simulink model "KinematicsSolverSimscape"  (R2018b)
settings: Solver=ode3  StartTime=0.0  StopTime=3  FixedStep=0.001  RelTol=1e-3
PreLoadFcn:
  | run('Arm6Assembly_DataFile.m');
model workspace: external: MAT-File E:\SixRobotArm\Simscape_Simulation\StepFile\Arm6Assembly_DataFile.mat (data not in the file)
values from neighbouring files (symbols this model uses):
  smiData =     [Arm6SimscapeData.mat]
undefined symbols (not defined in the file or in its folder): X, Y, Z
libraries: fl_lib x187, nesl_utility x55, sm_lib x36, elec_lib x12, simulink_extras x7, simulink x6
(part 1 of 4)
settings Model: Creator=Administrator  LastModifiedBy=Jeason
settings DataIOCC: ReturnWorkspaceOutputs=on
settings ExplorerConfigSet: InternalSimMechanicsExplorerSettings="<ExplorerConfiguration><canonicalview>planar_xy</canonicalview><AnimationSetting><BasePlaybackSpeed>1.0</BasePlaybackSpeed><PlaybackSpeedFactor>0.5</PlaybackSpeedFactor></AnimationSetting><TilePanel><TileInfo><Tiles Columns=\"1\" Count=\"1\" Rows=\"1\"><Column Weight=\"1\"/><Row Weight=\"1\"/><Tile Height=\"1\" Width=\"1\" X=\"0\" Y=\"0\"/></Tiles></TileInfo><SceneInfo><SceneViewer><BGColor><R>0.60000002384185791</R><G>0.60000002384185791</G><B>0.60000002384185791</B></BGColor><Camera><DoPerspective>off</DoPerspective><Position><X>-0.504262514033846698</X><Y>0.881384571408073469</Y><Z>0.0888981961479472504</Z></Position><Center><X>0.248760542540387375</X><Y>0.293287954006147933</Y><Z>-0.20622659926582132</Z></Center><Up><X>0.445605319462419325</X><Y>0.785803061090466048</Y><Z>-0.428893283285771199</Z></Up><ViewLimDist>1</ViewLimDist><YLim>0.601033807151443056</YLim><XLim>0.667231586610430694</XLim></Camera></SceneViewer></SceneInfo></TilePanel><MechEditorPanel><Cameras/><GfxPanelCameraMap/><VideoCreator><PlaybackSpeedRatio>1.0</PlaybackSpeedRatio><FrameRate>30</FrameRate><VideoFormat>MPEG-4</VideoFormat><FrameSize>[800 600]</FrameSize></VideoCreator></MechEditorPanel></ExplorerConfiguration>"

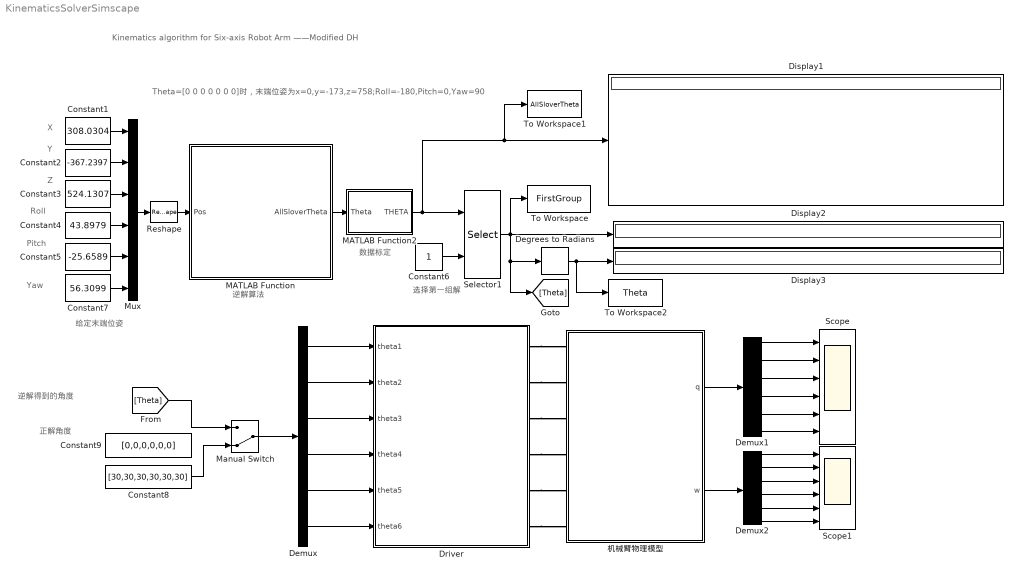
== system KinematicsSolverSimscape ==
  note: 选择第一组解
  note: 数据标定
  note: Kinematics algorithm for Six-axis Robot Arm ——Modified DH
  note: 正解角度
  note: Theta=[0 0 0 0 0 0 0]时，末端位姿为x=0,y=-173,z=758;Roll=-180,Pitch=0,Yaw=90
  note: 逆解得到的角度
  note: 逆解算法
  note: X
  note: Yaw
  note: 给定末端位姿
  note: Z
  note: Y
  note: Pitch
  note: Roll
  Constant1 : Constant  Value=308.0304
  Constant2 : Constant  Value=-367.2397
  Constant3 : Constant  Value=524.1307
  Constant4 : Constant  Value=43.8979
  Constant5 : Constant  Value=-25.6589
  Constant6 : Constant
  Constant7 : Constant  Value=56.3099
  Constant8 : Constant  Value=[30,30,30,30,30,30]
  Constant9 : Constant  Value=[0,0,0,0,0,0]
  Degrees to Radians : simulink_extras/Transformations/Degrees to Radians
  Demux : Demux  Outputs=6
  Demux1 : Demux  Outputs=6
  Demux2 : Demux  Outputs=6
  Display1 : Display
  Display2 : Display
  Display3 : Display
  Driver : Subsystem  mask{angle1=0, angle2=0, angle3=0, angle4=0, angle5=0, angle6=0}
      mask prompts: angle1 "InitTheta1(deg)"; angle2 "InitTheta2(deg)"; angle3 "InitTheta3(deg)"; angle4 "InitTheta4(deg)"; angle5 "InitTheta5(deg)"; angle6 "InitTheta6(deg)"
  MATLAB Function : MATLAB Function  TreatAsAtomicUnit=on
  MATLAB Function2 : MATLAB Function  TreatAsAtomicUnit=on
  Manual Switch : ManualSwitch  CurrentSetting=0
  Mux : Mux  Inputs=6
  Reshape : Reshape  OutputDimensionality=Customize  OutputDimensions=[1,6]
  Scope : Scope  NumInputPorts=6
  Scope1 : Scope  NumInputPorts=6
  Selector1 : Selector  NumberOfDimensions=2  InputPortWidth=10  IndexOptions=Index vector (port),Starting index (dialog)  Indices=[1 3],1  OutputSizes=1,6
  To Workspace : ToWorkspace  VariableName=FirstGroup  SampleTime=-1
      settings: MaxDataPoints=1
  To Workspace1 : ToWorkspace  VariableName=AllSloverTheta  SampleTime=-1
      settings: MaxDataPoints=1
  To Workspace2 : ToWorkspace  VariableName=Theta  SampleTime=-1
      settings: MaxDataPoints=1
  机械臂物理模型 : Subsystem
  wires:
  Constant2/1 -> Mux/2
  MATLAB Function2/1(THETA) -> To Workspace1/1, Display1/1, Selector1/1
  Constant1/1 -> Mux/1
  Demux/5 -> Driver/5(theta5)
  Constant7/1 -> Mux/6
  Manual Switch/1 -> Demux/1
  MATLAB Function/1(AllSloverTheta) -> MATLAB Function2/1(Theta)
  Demux/2 -> Driver/2(theta2)
  Mux/1 -> Reshape/1
  Constant6/1 -> Selector1/2
  Reshape/1 -> MATLAB Function/1(Pos)
  Demux/4 -> Driver/4(theta4)
  Degrees to Radians/1 -> To Workspace2/1, Display3/1
  Demux/3 -> Driver/3(theta3)
  [Theta] -> Manual Switch/1
  Selector1/1 -> To Workspace/1, [Theta], Degrees to Radians/1, Display2/1
  Constant3/1 -> Mux/3
  Demux/6 -> Driver/6(theta6)
  Constant4/1 -> Mux/4
  Constant5/1 -> Mux/5
  Demux/1 -> Driver/1(theta1)
  Constant8/1 -> Manual Switch/2
  机械臂物理模型/1(q) -> Demux1/1
  Demux1/1 -> Scope/1
  Demux1/2 -> Scope/2
  Demux1/3 -> Scope/3
  Demux1/4 -> Scope/4
  Demux1/5 -> Scope/5
  Demux1/6 -> Scope/6
  机械臂物理模型/2(w) -> Demux2/1
  Demux2/1 -> Scope1/1
  Demux2/2 -> Scope1/2
  Demux2/3 -> Scope1/3
  Demux2/4 -> Scope1/4
  Demux2/5 -> Scope1/5
  Demux2/6 -> Scope1/6
  connections:
  Driver/RConn1 -- 机械臂物理模型/LConn1
  Driver/RConn2 -- 机械臂物理模型/LConn2
  Driver/RConn3 -- 机械臂物理模型/LConn3
  Driver/RConn4 -- 机械臂物理模型/LConn4
  Driver/RConn5 -- 机械臂物理模型/LConn5
  Driver/RConn6 -- 机械臂物理模型/LConn6

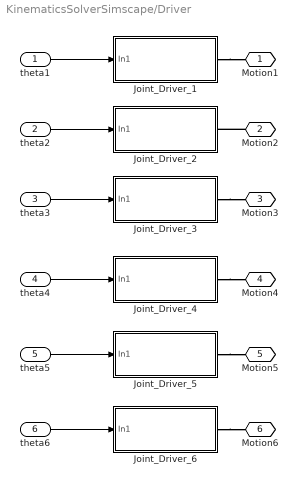
== system KinematicsSolverSimscape/Driver ==
  theta1 : Inport
  theta2 : Inport  Port=2
  theta3 : Inport  Port=3
  theta4 : Inport  Port=4
  theta5 : Inport  Port=5
  theta6 : Inport  Port=6
  Joint_Driver_1 : Subsystem
  Joint_Driver_2 : Subsystem
  Joint_Driver_3 : Subsystem
  Joint_Driver_4 : Subsystem
  Joint_Driver_5 : Subsystem
  Joint_Driver_6 : Subsystem
  Motion1 : PMIOPort  Side=Right
  Motion2 : PMIOPort  Port=2  Side=Right
  Motion3 : PMIOPort  Port=3  Side=Right
  Motion4 : PMIOPort  Port=4  Side=Right
  Motion5 : PMIOPort  Port=5  Side=Right
  Motion6 : PMIOPort  Port=6  Side=Right
  wires:
  theta5/1 -> Joint_Driver_5/1(In1)
  theta6/1 -> Joint_Driver_6/1(In1)
  theta4/1 -> Joint_Driver_4/1(In1)
  theta3/1 -> Joint_Driver_3/1(In1)
  theta2/1 -> Joint_Driver_2/1(In1)
  theta1/1 -> Joint_Driver_1/1(In1)
  connections:
  Joint_Driver_4/RConn1 -- Motion4/RConn1
  Joint_Driver_5/RConn1 -- Motion5/RConn1
  Joint_Driver_3/RConn1 -- Motion3/RConn1
  Joint_Driver_1/RConn1 -- Motion1/RConn1
  Joint_Driver_6/RConn1 -- Motion6/RConn1
  Motion2/RConn1 -- Joint_Driver_2/RConn1

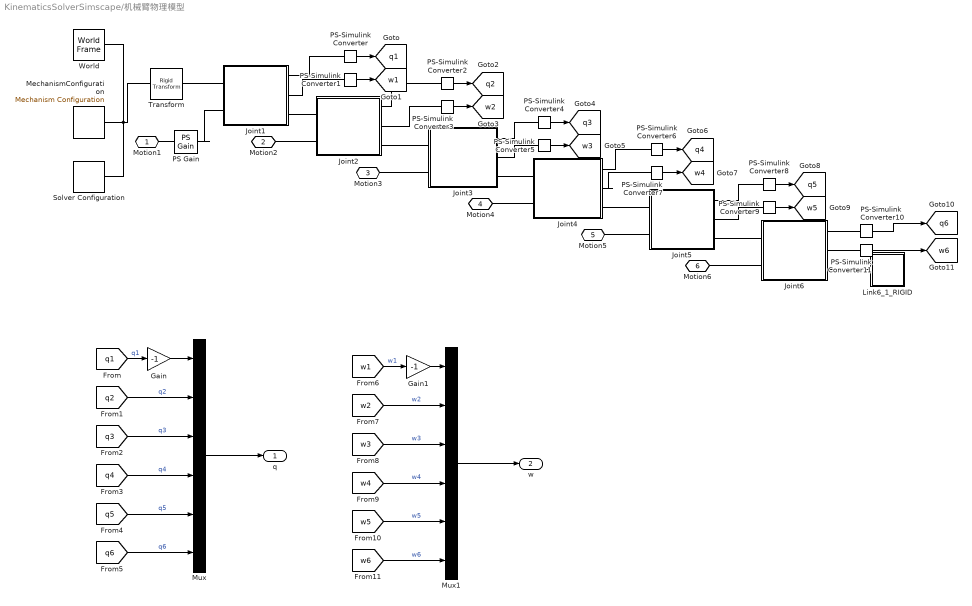
== system KinematicsSolverSimscape/机械臂物理模型 ==
  Gain : Gain  Gain=-1
  Gain1 : Gain  Gain=-1
  Joint1 : Subsystem
  Joint2 : Subsystem
  Joint3 : Subsystem
  Joint4 : Subsystem
  Joint5 : Subsystem
  Joint6 : Subsystem
  Link6_1_RIGID : Subsystem
  MechanismConfiguration : sm_lib/Utilities/Mechanism Configuration  UniformGravity=Constant  GravityVector=[0 -9.80665 0]  GravityUnits=m/s^2  LinearizationDelta=0.001
  Mux : Mux  Inputs=6
  Mux1 : Mux  Inputs=6
  PS Gain : fl_lib/Physical Signals/Functions/PS Gain  gain=-1
  PS-Simulink Converter{,2,4,6,8,10} (6 alike) : nesl_utility/PS-Simulink Converter  PhysicalDomain=network_engine_domain  SubClassName=ps_output  LeftPortType=input  RightPortType=output  PseudoPeriodic=off  Frequencies=[]  Unit=deg  AffineConversion=off
  PS-Simulink Converter{1,3,5,7,9,11} (6 alike) : nesl_utility/PS-Simulink Converter  PhysicalDomain=network_engine_domain  SubClassName=ps_output  LeftPortType=input  RightPortType=output  PseudoPeriodic=off  Frequencies=[]  Unit=deg/s  AffineConversion=off
  Solver Configuration : nesl_utility/Solver Configuration  PhysicalDomain=network_engine_domain  SubClassName=solver  LeftPortType=input  RightPortType=generic  Tones=[]  Harmonics=[]  SimulateNoise=off  Profile=off  UseLocalSampling=off  EnableSwitchedLinearOptims=on  FrequencyDomain=off  UseCCode=off  RelTol=0.001  AbsTol=1e-06  MinStep=1e-09  ToWorkspace=off  RevertToSquareIcSolve=off  NumHomotopyIterations=100  PhasorMode=off  PhasorModeNumHarmonics=1  DoDC=off  ResidualTolerance=1e-09  UseLocalSolver=off  LocalSolverChoice=NE_BACKWARD_EULER_ADVANCER  LocalSolverSampleTime=0.001  DoFixedCost=off  MaxNonlinIter=3  MaxModeIter=2  LinearAlgebra=auto  EquationFormulation=NE_TIME_EF  DelaysMemoryBudget=1024  AutomaticFiltering=on  FilteringTimeConstant=0.001  PartitionStorageMethod=AS_NEEDED  PartitionMemoryBudget=1024
  Transform : sm_lib/Frames and Transforms/Rigid Transform  TranslationMethod=Cartesian  TranslationStandardOffset=0  TranslationLengthUnit=mm  TranslationStandardAxis=+Z  TranslationCartesianOffset=smiData.RigidTransform(14).translation  TranslationROffset=0  TranslationROffsetUnits=m  TranslationZOffset=0  TranslationZOffsetUnits=m  TranslationThetaOffset=0  TranslationThetaOffsetUnits=deg  RotationMethod=ArbitraryAxis  RotationAngleUnits=rad  RotationStandardAxis=+Z  RotationAngle=smiData.RigidTransform(14).angle  RotationArbitraryAxis=smiData.RigidTransform(14).axis  FollAlignAxisA=+X  BaseAlignAxisA=+Y  FollAlignAxisB=+Y  BaseAlignAxisB=+Z  RotationSequenceAxes=FollowerAxes  RotationSequence=XYX  RotationSequenceAngles=[0 0 0]  RotationSequenceAnglesUnits=deg  RotationMatrix=[1 0 0; 0 1 0; 0 0 1]
  World : sm_lib/Frames and Transforms/World Frame
  Motion1 : PMIOPort  Side=Left
  Motion2 : PMIOPort  Port=2  Side=Left
  Motion3 : PMIOPort  Port=3  Side=Left
  Motion4 : PMIOPort  Port=4  Side=Left
  Motion5 : PMIOPort  Port=5  Side=Left
  Motion6 : PMIOPort  Port=6  Side=Left
  q : Outport  VectorParamsAs1DForOutWhenUnconnected=on
  w : Outport  Port=2  VectorParamsAs1DForOutWhenUnconnected=on
  tag scope: q1=global, q2=global, q3=global, q4=global, q5=global, q6=global, w1=global, w2=global, w3=global, w4=global, w5=global, w6=global
  wires:
  [q5] -> Mux/5  "q5"
  Mux/1 -> q/1
  PS-Simulink Converter6/1 -> [q4]
  [w4] -> Mux1/4  "w4"
  PS-Simulink Converter/1 -> [q1]
  [q6] -> Mux/6  "q6"
  [w1] -> Gain1/1  "w1"
  [w5] -> Mux1/5  "w5"
  PS-Simulink Converter4/1 -> [q3]
  PS-Simulink Converter5/1 -> [w3]
  PS-Simulink Converter9/1 -> [w5]
  [w2] -> Mux1/2  "w2"
  PS-Simulink Converter1/1 -> [w1]
  [q2] -> Mux/2  "q2"
  PS-Simulink Converter10/1 -> [q6]
  [w6] -> Mux1/6  "w6"
  PS-Simulink Converter7/1 -> [w4]
  [q4] -> Mux/4  "q4"
  PS-Simulink Converter11/1 -> [w6]
  PS-Simulink Converter8/1 -> [q5]
  Mux1/1 -> w/1
  PS-Simulink Converter2/1 -> [q2]
  [q3] -> Mux/3  "q3"
  [q1] -> Gain/1  "q1"
  [w3] -> Mux1/3  "w3"
  PS-Simulink Converter3/1 -> [w2]
  Gain/1 -> Mux/1
  Gain1/1 -> Mux1/1
  connections:
  Joint6/RConn1 -- PS-Simulink Converter10/LConn1
  PS-Simulink Converter11/LConn1 -- Joint6/RConn2
  Joint4/RConn2 -- PS-Simulink Converter7/LConn1
  Joint4/RConn1 -- PS-Simulink Converter6/LConn1
  PS-Simulink Converter9/LConn1 -- Joint5/RConn2
  PS-Simulink Converter5/LConn1 -- Joint3/RConn2
  Transform/LConn1 -- MechanismConfiguration/RConn1 -- Solver Configuration/RConn1 -- World/RConn1
  Joint3/RConn3 -- Joint4/LConn1
  Joint1/RConn2 -- PS-Simulink Converter1/LConn1
  PS-Simulink Converter3/LConn1 -- Joint2/RConn2
  Joint1/LConn1 -- Transform/RConn1
  PS-Simulink Converter8/LConn1 -- Joint5/RConn1
  Motion4/RConn1 -- Joint4/LConn2
  PS-Simulink Converter4/LConn1 -- Joint3/RConn1
  Joint1/RConn1 -- PS-Simulink Converter/LConn1
  Joint6/LConn1 -- Joint5/RConn3
  Joint3/LConn1 -- Joint2/RConn3
  Joint5/LConn1 -- Joint4/RConn3
  Link6_1_RIGID/LConn1 -- Joint6/RConn3
  Motion6/RConn1 -- Joint6/LConn2
  Motion2/RConn1 -- Joint2/LConn2
  PS-Simulink Converter2/LConn1 -- Joint2/RConn1
  Motion5/RConn1 -- Joint5/LConn2
  Joint2/LConn1 -- Joint1/RConn3
  Motion3/RConn1 -- Joint3/LConn2
  PS Gain/RConn1 -- Joint1/LConn2
  Motion1/RConn1 -- PS Gain/LConn1

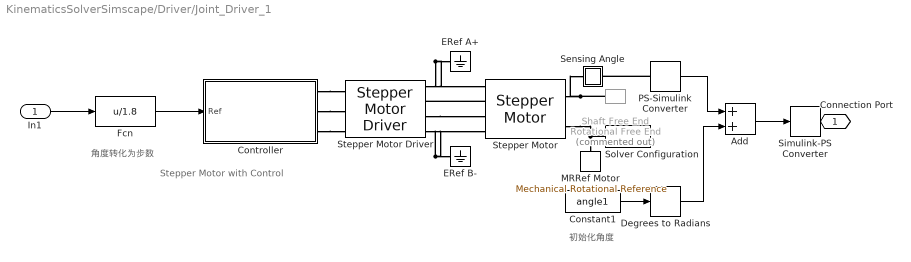
== system KinematicsSolverSimscape/Driver/Joint_Driver_1 ==
  note: 角度转化为步数
  note: Stepper Motor with Control
  note: 初始化角度
  In1 : Inport
  Add : Sum
  Constant1 : Constant  Value=angle1
  Controller : Subsystem  VariantControlMode=Label  Variant=on  LabelModeActiveChoice=Position
      settings: AttributesFormatString=%<BlockChoice>
  Degrees to Radians : simulink_extras/Transformations/Degrees to Radians
  ERef A+ : fl_lib/Electrical/Electrical Elements/Electrical Reference
      settings: SourceProductName=Foundation Library
  ERef B- : fl_lib/Electrical/Electrical Elements/Electrical Reference
      settings: SourceProductName=Foundation Library
  Fcn : Fcn  Expr=u/1.8
  MRRef Motor : fl_lib/Mechanical/Rotational Elements/Mechanical Rotational Reference
      settings: SourceProductName=Foundation Library
  PS-Simulink Converter : nesl_utility/PS-Simulink Converter  PhysicalDomain=network_engine_domain  SubClassName=ps_output  LeftPortType=input  RightPortType=output  PseudoPeriodic=off  Frequencies=[]  Unit=1  AffineConversion=off
  Sensing Angle : Subsystem
      mask Display: disp('a')
  Shaft Free End : fl_lib/Mechanical/Rotational Elements/Rotational Free End  Commented=on  w_specify=off  w_priority=None  w=0 rad/s  w_nominal_specify=off  w_nominal_unit=rad/s  w_nominal_value=1
      settings: SourceProductName=Foundation Library
  Simulink-PS Converter : nesl_utility/Simulink-PS Converter  PhysicalDomain=network_engine_domain  SubClassName=ps_input  LeftPortType=input  RightPortType=output  PseudoPeriodic=off  Frequencies=[]  NoiseDistribution=none  NoiseParameters=[]  Unit=1  AffineConversion=off  FilteringAndDerivatives=provide  SimscapeFilterOrder=2  InputFilterTimeConstant=0.001  UdotUserProvided=0
  Solver Configuration : nesl_utility/Solver Configuration  PhysicalDomain=network_engine_domain  SubClassName=solver  LeftPortType=input  RightPortType=generic  Tones=[]  Harmonics=[]  SimulateNoise=off  Profile=off  UseLocalSampling=off  EnableSwitchedLinearOptims=on  FrequencyDomain=off  UseCCode=off  RelTol=0.001  AbsTol=1e-06  MinStep=1e-09  ToWorkspace=off  RevertToSquareIcSolve=off  NumHomotopyIterations=100  PhasorMode=off  PhasorModeNumHarmonics=1  DoDC=off  ResidualTolerance=1e-9  UseLocalSolver=off  LocalSolverChoice=NE_BACKWARD_EULER_ADVANCER  LocalSolverSampleTime=.001  DoFixedCost=off  MaxNonlinIter=3  MaxModeIter=2  LinearAlgebra=Sparse  EquationFormulation=NE_TIME_EF  DelaysMemoryBudget=1024  AutomaticFiltering=on  FilteringTimeConstant=0.001  PartitionStorageMethod=AS_NEEDED  PartitionMemoryBudget=1024
  Stepper Motor : elec_lib/Actuators & Drivers/Rotational Actuators/Stepper Motor  step_or_av=1  w_vec=[ 0 1000 3e+3 ] rpm  T_vec=[ 2 2 1 ] N*m  assert_if_slipping=0  J_total=1e-4 kg*m^2  max_step_rate=10 Hz  Ra=0.55 Ohm  La=0.0015 H  Km=0.19 N*m/A  Td=0 N*m  Rm=Inf Ohm  Step=1.8 deg  J=4.5e-05 kg*m^2  B=1e-02 N*m/(rad/s)  speed0=0 rpm  theta0=0 deg  alpha=[ 0.00393 0.00393 ] 1/K  Tmeas=25 degC  T_vec2=[ 1.7 1.7 0.85 ] N*m  Tmeas2=125 degC  half_stepping=0  thermal_masses=[ 100 100 ] J/K  initial_temperatures=[ 25 25 ] degC  rotor_thermal_mass=50 J/K  rotor_initial_temperature=25 degC  Rm_percent_rotor=90
      settings: SourceProductName=Simscape Electronics  SourceProductBaseCode=SN
  Stepper Motor Driver : elec_lib/Actuators & Drivers/Drivers/Stepper Motor Driver  step_or_av=1  step_rate_per_volt=10 Hz/V  Venable=2.5 V  Vreverse=2.5 V  Vm=5 V  half_stepping=0
      settings: SourceProductName=Simscape Electronics  SourceProductBaseCode=SN
  Connection Port : PMIOPort  Side=Right
  wires:
  Degrees to Radians/1 -> Add/2
  Add/1 -> Simulink-PS Converter/1
  PS-Simulink Converter/1 -> Add/1
  Constant1/1 -> Degrees to Radians/1
  In1/1 -> Fcn/1
  Fcn/1 -> Controller/1(Ref)
  connections:
  Connection Port/RConn1 -- Simulink-PS Converter/RConn1
  ERef B-/LConn1 -- Stepper Motor Driver/RConn4 -- Stepper Motor/LConn4
  Stepper Motor/RConn1 -- Sensing Angle/LConn1 -- Shaft Free End/LConn1
  MRRef Motor/LConn1 -- Stepper Motor/RConn2 -- Solver Configuration/RConn1
  ERef A+/LConn1 -- Stepper Motor Driver/RConn1 -- Stepper Motor/LConn1
  Stepper Motor Driver/RConn3 -- Stepper Motor/LConn3
  Stepper Motor/LConn2 -- Stepper Motor Driver/RConn2
  Controller/RConn1 -- Stepper Motor Driver/LConn1
  Controller/RConn2 -- Stepper Motor Driver/LConn2
  Controller/RConn3 -- Stepper Motor Driver/LConn3
  PS-Simulink Converter/LConn1 -- Sensing Angle/RConn1

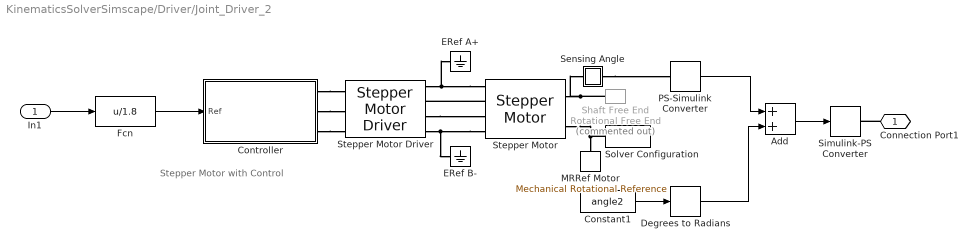
== system KinematicsSolverSimscape/Driver/Joint_Driver_2 ==
  note: Stepper Motor with Control
  In1 : Inport
  Add : Sum
  Constant1 : Constant  Value=angle2
  Controller : Subsystem  VariantControlMode=Label  Variant=on  LabelModeActiveChoice=Position
      settings: AttributesFormatString=%<BlockChoice>
  Degrees to Radians : simulink_extras/Transformations/Degrees to Radians
  ERef A+ : fl_lib/Electrical/Electrical Elements/Electrical Reference
      settings: SourceProductName=Foundation Library
  ERef B- : fl_lib/Electrical/Electrical Elements/Electrical Reference
      settings: SourceProductName=Foundation Library
  Fcn : Fcn  Expr=u/1.8
  MRRef Motor : fl_lib/Mechanical/Rotational Elements/Mechanical Rotational Reference
      settings: SourceProductName=Foundation Library
  PS-Simulink Converter : nesl_utility/PS-Simulink Converter  PhysicalDomain=network_engine_domain  SubClassName=ps_output  LeftPortType=input  RightPortType=output  PseudoPeriodic=off  Frequencies=[]  Unit=1  AffineConversion=off
  Sensing Angle : Subsystem
      mask Display: disp('a')
  Shaft Free End : fl_lib/Mechanical/Rotational Elements/Rotational Free End  Commented=on  w_specify=off  w_priority=None  w=0 rad/s  w_nominal_specify=off  w_nominal_unit=rad/s  w_nominal_value=1
      settings: SourceProductName=Foundation Library
  Simulink-PS Converter : nesl_utility/Simulink-PS Converter  PhysicalDomain=network_engine_domain  SubClassName=ps_input  LeftPortType=input  RightPortType=output  PseudoPeriodic=off  Frequencies=[]  NoiseDistribution=none  NoiseParameters=[]  Unit=1  AffineConversion=off  FilteringAndDerivatives=provide  SimscapeFilterOrder=2  InputFilterTimeConstant=0.001  UdotUserProvided=0
  Solver Configuration : nesl_utility/Solver Configuration  PhysicalDomain=network_engine_domain  SubClassName=solver  LeftPortType=input  RightPortType=generic  Tones=[]  Harmonics=[]  SimulateNoise=off  Profile=off  UseLocalSampling=off  EnableSwitchedLinearOptims=on  FrequencyDomain=off  UseCCode=off  RelTol=0.001  AbsTol=1e-06  MinStep=1e-09  ToWorkspace=off  RevertToSquareIcSolve=off  NumHomotopyIterations=100  PhasorMode=off  PhasorModeNumHarmonics=1  DoDC=off  ResidualTolerance=1e-9  UseLocalSolver=off  LocalSolverChoice=NE_BACKWARD_EULER_ADVANCER  LocalSolverSampleTime=.001  DoFixedCost=off  MaxNonlinIter=3  MaxModeIter=2  LinearAlgebra=Sparse  EquationFormulation=NE_TIME_EF  DelaysMemoryBudget=1024  AutomaticFiltering=on  FilteringTimeConstant=0.001  PartitionStorageMethod=AS_NEEDED  PartitionMemoryBudget=1024
  Stepper Motor : elec_lib/Actuators & Drivers/Rotational Actuators/Stepper Motor  step_or_av=1  w_vec=[ 0 1000 3e+3 ] rpm  T_vec=[ 2 2 1 ] N*m  assert_if_slipping=0  J_total=1e-4 kg*m^2  max_step_rate=10 Hz  Ra=0.55 Ohm  La=0.0015 H  Km=0.19 N*m/A  Td=0 N*m  Rm=Inf Ohm  Step=1.8 deg  J=4.5e-05 kg*m^2  B=1e-02 N*m/(rad/s)  speed0=0 rpm  theta0=0 deg  alpha=[ 0.00393 0.00393 ] 1/K  Tmeas=25 degC  T_vec2=[ 1.7 1.7 0.85 ] N*m  Tmeas2=125 degC  half_stepping=0  thermal_masses=[ 100 100 ] J/K  initial_temperatures=[ 25 25 ] degC  rotor_thermal_mass=50 J/K  rotor_initial_temperature=25 degC  Rm_percent_rotor=90
      settings: SourceProductName=Simscape Electronics  SourceProductBaseCode=SN
  Stepper Motor Driver : elec_lib/Actuators & Drivers/Drivers/Stepper Motor Driver  step_or_av=1  step_rate_per_volt=10 Hz/V  Venable=2.5 V  Vreverse=2.5 V  Vm=5 V  half_stepping=0
      settings: SourceProductName=Simscape Electronics  SourceProductBaseCode=SN
  Connection Port1 : PMIOPort  Side=Right
  wires:
  Degrees to Radians/1 -> Add/2
  PS-Simulink Converter/1 -> Add/1
  Constant1/1 -> Degrees to Radians/1
  Add/1 -> Simulink-PS Converter/1
  Fcn/1 -> Controller/1(Ref)
  In1/1 -> Fcn/1
  connections:
  Connection Port1/RConn1 -- Simulink-PS Converter/RConn1
  Sensing Angle/RConn1 -- PS-Simulink Converter/LConn1
  Controller/RConn3 -- Stepper Motor Driver/LConn3
  Controller/RConn2 -- Stepper Motor Driver/LConn2
  Controller/RConn1 -- Stepper Motor Driver/LConn1
  Stepper Motor/LConn2 -- Stepper Motor Driver/RConn2
  Stepper Motor Driver/RConn3 -- Stepper Motor/LConn3
  Stepper Motor/LConn1 -- Stepper Motor Driver/RConn1 -- ERef A+/LConn1
  Solver Configuration/RConn1 -- Stepper Motor/RConn2 -- MRRef Motor/LConn1
  Stepper Motor/RConn1 -- Shaft Free End/LConn1 -- Sensing Angle/LConn1
  Stepper Motor/LConn4 -- Stepper Motor Driver/RConn4 -- ERef B-/LConn1

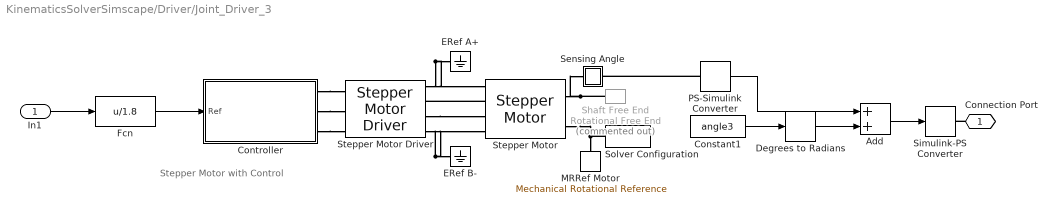
== system KinematicsSolverSimscape/Driver/Joint_Driver_3 ==
  note: Stepper Motor with Control
  In1 : Inport
  Add : Sum
  Constant1 : Constant  Value=angle3
  Controller : Subsystem  VariantControlMode=Label  Variant=on  LabelModeActiveChoice=Position
      settings: AttributesFormatString=%<BlockChoice>
  Degrees to Radians : simulink_extras/Transformations/Degrees to Radians
  ERef A+ : fl_lib/Electrical/Electrical Elements/Electrical Reference
      settings: SourceProductName=Foundation Library
  ERef B- : fl_lib/Electrical/Electrical Elements/Electrical Reference
      settings: SourceProductName=Foundation Library
  Fcn : Fcn  Expr=u/1.8
  MRRef Motor : fl_lib/Mechanical/Rotational Elements/Mechanical Rotational Reference
      settings: SourceProductName=Foundation Library
  PS-Simulink Converter : nesl_utility/PS-Simulink Converter  PhysicalDomain=network_engine_domain  SubClassName=ps_output  LeftPortType=input  RightPortType=output  PseudoPeriodic=off  Frequencies=[]  Unit=1  AffineConversion=off
  Sensing Angle : Subsystem
      mask Display: disp('a')
  Shaft Free End : fl_lib/Mechanical/Rotational Elements/Rotational Free End  Commented=on  w_specify=off  w_priority=None  w=0 rad/s  w_nominal_specify=off  w_nominal_unit=rad/s  w_nominal_value=1
      settings: SourceProductName=Foundation Library
  Simulink-PS Converter : nesl_utility/Simulink-PS Converter  PhysicalDomain=network_engine_domain  SubClassName=ps_input  LeftPortType=input  RightPortType=output  PseudoPeriodic=off  Frequencies=[]  NoiseDistribution=none  NoiseParameters=[]  Unit=1  AffineConversion=off  FilteringAndDerivatives=provide  SimscapeFilterOrder=2  InputFilterTimeConstant=0.001  UdotUserProvided=0
  Solver Configuration : nesl_utility/Solver Configuration  PhysicalDomain=network_engine_domain  SubClassName=solver  LeftPortType=input  RightPortType=generic  Tones=[]  Harmonics=[]  SimulateNoise=off  Profile=off  UseLocalSampling=off  EnableSwitchedLinearOptims=on  FrequencyDomain=off  UseCCode=off  RelTol=0.001  AbsTol=1e-06  MinStep=1e-09  ToWorkspace=off  RevertToSquareIcSolve=off  NumHomotopyIterations=100  PhasorMode=off  PhasorModeNumHarmonics=1  DoDC=off  ResidualTolerance=1e-9  UseLocalSolver=off  LocalSolverChoice=NE_BACKWARD_EULER_ADVANCER  LocalSolverSampleTime=.001  DoFixedCost=off  MaxNonlinIter=3  MaxModeIter=2  LinearAlgebra=Sparse  EquationFormulation=NE_TIME_EF  DelaysMemoryBudget=1024  AutomaticFiltering=on  FilteringTimeConstant=0.001  PartitionStorageMethod=AS_NEEDED  PartitionMemoryBudget=1024
  Stepper Motor : elec_lib/Actuators & Drivers/Rotational Actuators/Stepper Motor  step_or_av=1  w_vec=[ 0 1000 3e+3 ] rpm  T_vec=[ 2 2 1 ] N*m  assert_if_slipping=0  J_total=1e-4 kg*m^2  max_step_rate=10 Hz  Ra=0.55 Ohm  La=0.0015 H  Km=0.19 N*m/A  Td=0 N*m  Rm=Inf Ohm  Step=1.8 deg  J=4.5e-05 kg*m^2  B=1e-02 N*m/(rad/s)  speed0=0 rpm  theta0=0 deg  alpha=[ 0.00393 0.00393 ] 1/K  Tmeas=25 degC  T_vec2=[ 1.7 1.7 0.85 ] N*m  Tmeas2=125 degC  half_stepping=0  thermal_masses=[ 100 100 ] J/K  initial_temperatures=[ 25 25 ] degC  rotor_thermal_mass=50 J/K  rotor_initial_temperature=25 degC  Rm_percent_rotor=90
      settings: SourceProductName=Simscape Electronics  SourceProductBaseCode=SN
  Stepper Motor Driver : elec_lib/Actuators & Drivers/Drivers/Stepper Motor Driver  step_or_av=1  step_rate_per_volt=10 Hz/V  Venable=2.5 V  Vreverse=2.5 V  Vm=5 V  half_stepping=0
      settings: SourceProductName=Simscape Electronics  SourceProductBaseCode=SN
  Connection Port : PMIOPort  Side=Right
  wires:
  Degrees to Radians/1 -> Add/2
  PS-Simulink Converter/1 -> Add/1
  Constant1/1 -> Degrees to Radians/1
  Add/1 -> Simulink-PS Converter/1
  In1/1 -> Fcn/1
  Fcn/1 -> Controller/1(Ref)
  connections:
  Connection Port/RConn1 -- Simulink-PS Converter/RConn1
  ERef B-/LConn1 -- Stepper Motor Driver/RConn4 -- Stepper Motor/LConn4
  Stepper Motor/RConn1 -- Sensing Angle/LConn1 -- Shaft Free End/LConn1
  MRRef Motor/LConn1 -- Stepper Motor/RConn2 -- Solver Configuration/RConn1
  ERef A+/LConn1 -- Stepper Motor Driver/RConn1 -- Stepper Motor/LConn1
  Stepper Motor Driver/RConn3 -- Stepper Motor/LConn3
  Stepper Motor/LConn2 -- Stepper Motor Driver/RConn2
  Controller/RConn1 -- Stepper Motor Driver/LConn1
  Controller/RConn2 -- Stepper Motor Driver/LConn2
  Controller/RConn3 -- Stepper Motor Driver/LConn3
  PS-Simulink Converter/LConn1 -- Sensing Angle/RConn1

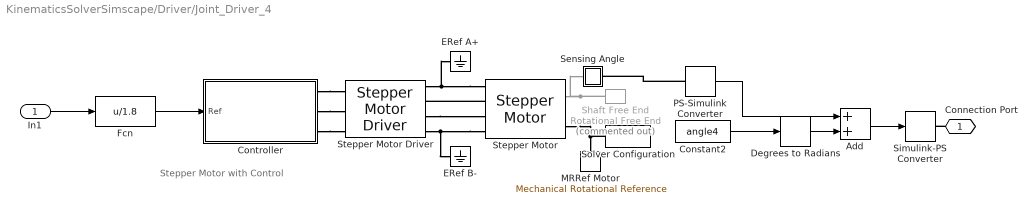
== system KinematicsSolverSimscape/Driver/Joint_Driver_4 ==
  note: Stepper Motor with Control
  In1 : Inport
  Add : Sum
  Constant2 : Constant  Value=angle4
  Controller : Subsystem  VariantControlMode=Label  Variant=on  LabelModeActiveChoice=Position
      settings: AttributesFormatString=%<BlockChoice>
  Degrees to Radians : simulink_extras/Transformations/Degrees to Radians
  ERef A+ : fl_lib/Electrical/Electrical Elements/Electrical Reference
      settings: SourceProductName=Foundation Library
  ERef B- : fl_lib/Electrical/Electrical Elements/Electrical Reference
      settings: SourceProductName=Foundation Library
  Fcn : Fcn  Expr=u/1.8
  MRRef Motor : fl_lib/Mechanical/Rotational Elements/Mechanical Rotational Reference
      settings: SourceProductName=Foundation Library
  PS-Simulink Converter : nesl_utility/PS-Simulink Converter  PhysicalDomain=network_engine_domain  SubClassName=ps_output  LeftPortType=input  RightPortType=output  PseudoPeriodic=off  Frequencies=[]  Unit=1  AffineConversion=off
  Sensing Angle : Subsystem
      mask Display: disp('a')
  Shaft Free End : fl_lib/Mechanical/Rotational Elements/Rotational Free End  Commented=on  w_specify=off  w_priority=None  w=0 rad/s  w_nominal_specify=off  w_nominal_unit=rad/s  w_nominal_value=1
      settings: SourceProductName=Foundation Library
  Simulink-PS Converter : nesl_utility/Simulink-PS Converter  PhysicalDomain=network_engine_domain  SubClassName=ps_input  LeftPortType=input  RightPortType=output  PseudoPeriodic=off  Frequencies=[]  NoiseDistribution=none  NoiseParameters=[]  Unit=1  AffineConversion=off  FilteringAndDerivatives=provide  SimscapeFilterOrder=2  InputFilterTimeConstant=0.001  UdotUserProvided=0
  Solver Configuration : nesl_utility/Solver Configuration  PhysicalDomain=network_engine_domain  SubClassName=solver  LeftPortType=input  RightPortType=generic  Tones=[]  Harmonics=[]  SimulateNoise=off  Profile=off  UseLocalSampling=off  EnableSwitchedLinearOptims=on  FrequencyDomain=off  UseCCode=off  RelTol=0.001  AbsTol=1e-06  MinStep=1e-09  ToWorkspace=off  RevertToSquareIcSolve=off  NumHomotopyIterations=100  PhasorMode=off  PhasorModeNumHarmonics=1  DoDC=off  ResidualTolerance=1e-9  UseLocalSolver=off  LocalSolverChoice=NE_BACKWARD_EULER_ADVANCER  LocalSolverSampleTime=.001  DoFixedCost=off  MaxNonlinIter=3  MaxModeIter=2  LinearAlgebra=Sparse  EquationFormulation=NE_TIME_EF  DelaysMemoryBudget=1024  AutomaticFiltering=on  FilteringTimeConstant=0.001  PartitionStorageMethod=AS_NEEDED  PartitionMemoryBudget=1024
  Stepper Motor : elec_lib/Actuators & Drivers/Rotational Actuators/Stepper Motor  step_or_av=1  w_vec=[ 0 1000 3e+3 ] rpm  T_vec=[ 2 2 1 ] N*m  assert_if_slipping=0  J_total=1e-4 kg*m^2  max_step_rate=10 Hz  Ra=0.55 Ohm  La=0.0015 H  Km=0.19 N*m/A  Td=0 N*m  Rm=Inf Ohm  Step=1.8 deg  J=4.5e-05 kg*m^2  B=1e-02 N*m/(rad/s)  speed0=0 rpm  theta0=0 deg  alpha=[ 0.00393 0.00393 ] 1/K  Tmeas=25 degC  T_vec2=[ 1.7 1.7 0.85 ] N*m  Tmeas2=125 degC  half_stepping=0  thermal_masses=[ 100 100 ] J/K  initial_temperatures=[ 25 25 ] degC  rotor_thermal_mass=50 J/K  rotor_initial_temperature=25 degC  Rm_percent_rotor=90
      settings: SourceProductName=Simscape Electronics  SourceProductBaseCode=SN
  Stepper Motor Driver : elec_lib/Actuators & Drivers/Drivers/Stepper Motor Driver  step_or_av=1  step_rate_per_volt=10 Hz/V  Venable=2.5 V  Vreverse=2.5 V  Vm=5 V  half_stepping=0
      settings: SourceProductName=Simscape Electronics  SourceProductBaseCode=SN
  Connection Port : PMIOPort  Side=Right
  wires:
  Degrees to Radians/1 -> Add/2
  PS-Simulink Converter/1 -> Add/1
  Constant2/1 -> Degrees to Radians/1
  Add/1 -> Simulink-PS Converter/1
  Fcn/1 -> Controller/1(Ref)
  In1/1 -> Fcn/1
  connections:
  Connection Port/RConn1 -- Simulink-PS Converter/RConn1
  PS-Simulink Converter/LConn1 -- Sensing Angle/RConn1
  Controller/RConn3 -- Stepper Motor Driver/LConn3
  Controller/RConn2 -- Stepper Motor Driver/LConn2
  Controller/RConn1 -- Stepper Motor Driver/LConn1
  Stepper Motor/LConn2 -- Stepper Motor Driver/RConn2
  Stepper Motor Driver/RConn3 -- Stepper Motor/LConn3
  Stepper Motor/LConn1 -- Stepper Motor Driver/RConn1 -- ERef A+/LConn1
  Solver Configuration/RConn1 -- Stepper Motor/RConn2 -- MRRef Motor/LConn1
  Shaft Free End/LConn1 -- Sensing Angle/LConn1 -- Stepper Motor/RConn1
  Stepper Motor/LConn4 -- Stepper Motor Driver/RConn4 -- ERef B-/LConn1

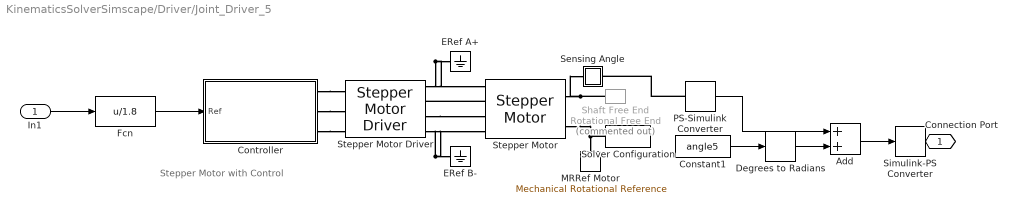
== system KinematicsSolverSimscape/Driver/Joint_Driver_5 ==
  note: Stepper Motor with Control
  In1 : Inport
  Add : Sum
  Constant1 : Constant  Value=angle5
  Controller : Subsystem  VariantControlMode=Label  Variant=on  LabelModeActiveChoice=Position
      settings: AttributesFormatString=%<BlockChoice>
  Degrees to Radians : simulink_extras/Transformations/Degrees to Radians
  ERef A+ : fl_lib/Electrical/Electrical Elements/Electrical Reference
      settings: SourceProductName=Foundation Library
  ERef B- : fl_lib/Electrical/Electrical Elements/Electrical Reference
      settings: SourceProductName=Foundation Library
  Fcn : Fcn  Expr=u/1.8
  MRRef Motor : fl_lib/Mechanical/Rotational Elements/Mechanical Rotational Reference
      settings: SourceProductName=Foundation Library
  PS-Simulink Converter : nesl_utility/PS-Simulink Converter  PhysicalDomain=network_engine_domain  SubClassName=ps_output  LeftPortType=input  RightPortType=output  PseudoPeriodic=off  Frequencies=[]  Unit=1  AffineConversion=off
  Sensing Angle : Subsystem
      mask Display: disp('a')
  Shaft Free End : fl_lib/Mechanical/Rotational Elements/Rotational Free End  Commented=on  w_specify=off  w_priority=None  w=0 rad/s  w_nominal_specify=off  w_nominal_unit=rad/s  w_nominal_value=1
      settings: SourceProductName=Foundation Library
  Simulink-PS Converter : nesl_utility/Simulink-PS Converter  PhysicalDomain=network_engine_domain  SubClassName=ps_input  LeftPortType=input  RightPortType=output  PseudoPeriodic=off  Frequencies=[]  NoiseDistribution=none  NoiseParameters=[]  Unit=1  AffineConversion=off  FilteringAndDerivatives=provide  SimscapeFilterOrder=2  InputFilterTimeConstant=0.001  UdotUserProvided=0
  Solver Configuration : nesl_utility/Solver Configuration  PhysicalDomain=network_engine_domain  SubClassName=solver  LeftPortType=input  RightPortType=generic  Tones=[]  Harmonics=[]  SimulateNoise=off  Profile=off  UseLocalSampling=off  EnableSwitchedLinearOptims=on  FrequencyDomain=off  UseCCode=off  RelTol=0.001  AbsTol=1e-06  MinStep=1e-09  ToWorkspace=off  RevertToSquareIcSolve=off  NumHomotopyIterations=100  PhasorMode=off  PhasorModeNumHarmonics=1  DoDC=off  ResidualTolerance=1e-9  UseLocalSolver=off  LocalSolverChoice=NE_BACKWARD_EULER_ADVANCER  LocalSolverSampleTime=.001  DoFixedCost=off  MaxNonlinIter=3  MaxModeIter=2  LinearAlgebra=Sparse  EquationFormulation=NE_TIME_EF  DelaysMemoryBudget=1024  AutomaticFiltering=on  FilteringTimeConstant=0.001  PartitionStorageMethod=AS_NEEDED  PartitionMemoryBudget=1024
  Stepper Motor : elec_lib/Actuators & Drivers/Rotational Actuators/Stepper Motor  step_or_av=1  w_vec=[ 0 1000 3e+3 ] rpm  T_vec=[ 2 2 1 ] N*m  assert_if_slipping=0  J_total=1e-4 kg*m^2  max_step_rate=10 Hz  Ra=0.55 Ohm  La=0.0015 H  Km=0.19 N*m/A  Td=0 N*m  Rm=Inf Ohm  Step=1.8 deg  J=4.5e-05 kg*m^2  B=1e-02 N*m/(rad/s)  speed0=0 rpm  theta0=0 deg  alpha=[ 0.00393 0.00393 ] 1/K  Tmeas=25 degC  T_vec2=[ 1.7 1.7 0.85 ] N*m  Tmeas2=125 degC  half_stepping=0  thermal_masses=[ 100 100 ] J/K  initial_temperatures=[ 25 25 ] degC  rotor_thermal_mass=50 J/K  rotor_initial_temperature=25 degC  Rm_percent_rotor=90
      settings: SourceProductName=Simscape Electronics  SourceProductBaseCode=SN
  Stepper Motor Driver : elec_lib/Actuators & Drivers/Drivers/Stepper Motor Driver  step_or_av=1  step_rate_per_volt=10 Hz/V  Venable=2.5 V  Vreverse=2.5 V  Vm=5 V  half_stepping=0
      settings: SourceProductName=Simscape Electronics  SourceProductBaseCode=SN
  Connection Port : PMIOPort  Side=Right
  wires:
  Degrees to Radians/1 -> Add/2
  PS-Simulink Converter/1 -> Add/1
  Constant1/1 -> Degrees to Radians/1
  Add/1 -> Simulink-PS Converter/1
  In1/1 -> Fcn/1
  Fcn/1 -> Controller/1(Ref)
  connections:
  Connection Port/RConn1 -- Simulink-PS Converter/RConn1
  ERef B-/LConn1 -- Stepper Motor Driver/RConn4 -- Stepper Motor/LConn4
  Stepper Motor/RConn1 -- Sensing Angle/LConn1 -- Shaft Free End/LConn1
  MRRef Motor/LConn1 -- Stepper Motor/RConn2 -- Solver Configuration/RConn1
  ERef A+/LConn1 -- Stepper Motor Driver/RConn1 -- Stepper Motor/LConn1
  Stepper Motor Driver/RConn3 -- Stepper Motor/LConn3
  Stepper Motor/LConn2 -- Stepper Motor Driver/RConn2
  Controller/RConn1 -- Stepper Motor Driver/LConn1
  Controller/RConn2 -- Stepper Motor Driver/LConn2
  Controller/RConn3 -- Stepper Motor Driver/LConn3
  PS-Simulink Converter/LConn1 -- Sensing Angle/RConn1

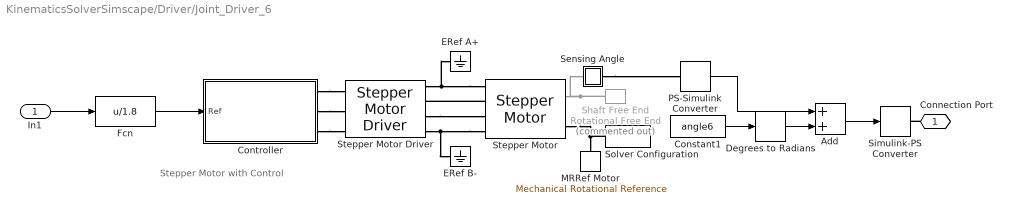
== system KinematicsSolverSimscape/Driver/Joint_Driver_6 ==
  note: Stepper Motor with Control
  In1 : Inport
  Add : Sum
  Constant1 : Constant  Value=angle6
  Controller : Subsystem  VariantControlMode=Label  Variant=on  LabelModeActiveChoice=Position
      settings: AttributesFormatString=%<BlockChoice>
  Degrees to Radians : simulink_extras/Transformations/Degrees to Radians
  ERef A+ : fl_lib/Electrical/Electrical Elements/Electrical Reference
      settings: SourceProductName=Foundation Library
  ERef B- : fl_lib/Electrical/Electrical Elements/Electrical Reference
      settings: SourceProductName=Foundation Library
  Fcn : Fcn  Expr=u/1.8
  MRRef Motor : fl_lib/Mechanical/Rotational Elements/Mechanical Rotational Reference
      settings: SourceProductName=Foundation Library
  PS-Simulink Converter : nesl_utility/PS-Simulink Converter  PhysicalDomain=network_engine_domain  SubClassName=ps_output  LeftPortType=input  RightPortType=output  PseudoPeriodic=off  Frequencies=[]  Unit=1  AffineConversion=off
  Sensing Angle : Subsystem
      mask Display: disp('a')
  Shaft Free End : fl_lib/Mechanical/Rotational Elements/Rotational Free End  Commented=on  w_specify=off  w_priority=None  w=0 rad/s  w_nominal_specify=off  w_nominal_unit=rad/s  w_nominal_value=1
      settings: SourceProductName=Foundation Library
  Simulink-PS Converter : nesl_utility/Simulink-PS Converter  PhysicalDomain=network_engine_domain  SubClassName=ps_input  LeftPortType=input  RightPortType=output  PseudoPeriodic=off  Frequencies=[]  NoiseDistribution=none  NoiseParameters=[]  Unit=1  AffineConversion=off  FilteringAndDerivatives=provide  SimscapeFilterOrder=2  InputFilterTimeConstant=0.001  UdotUserProvided=0
  Solver Configuration : nesl_utility/Solver Configuration  PhysicalDomain=network_engine_domain  SubClassName=solver  LeftPortType=input  RightPortType=generic  Tones=[]  Harmonics=[]  SimulateNoise=off  Profile=off  UseLocalSampling=off  EnableSwitchedLinearOptims=on  FrequencyDomain=off  UseCCode=off  RelTol=0.001  AbsTol=1e-06  MinStep=1e-09  ToWorkspace=off  RevertToSquareIcSolve=off  NumHomotopyIterations=100  PhasorMode=off  PhasorModeNumHarmonics=1  DoDC=off  ResidualTolerance=1e-9  UseLocalSolver=off  LocalSolverChoice=NE_BACKWARD_EULER_ADVANCER  LocalSolverSampleTime=.001  DoFixedCost=off  MaxNonlinIter=3  MaxModeIter=2  LinearAlgebra=Sparse  EquationFormulation=NE_TIME_EF  DelaysMemoryBudget=1024  AutomaticFiltering=on  FilteringTimeConstant=0.001  PartitionStorageMethod=AS_NEEDED  PartitionMemoryBudget=1024
  Stepper Motor : elec_lib/Actuators & Drivers/Rotational Actuators/Stepper Motor  step_or_av=1  w_vec=[ 0 1000 3e+3 ] rpm  T_vec=[ 2 2 1 ] N*m  assert_if_slipping=0  J_total=1e-4 kg*m^2  max_step_rate=10 Hz  Ra=0.55 Ohm  La=0.0015 H  Km=0.19 N*m/A  Td=0 N*m  Rm=Inf Ohm  Step=1.8 deg  J=4.5e-05 kg*m^2  B=1e-02 N*m/(rad/s)  speed0=0 rpm  theta0=0 deg  alpha=[ 0.00393 0.00393 ] 1/K  Tmeas=25 degC  T_vec2=[ 1.7 1.7 0.85 ] N*m  Tmeas2=125 degC  half_stepping=0  thermal_masses=[ 100 100 ] J/K  initial_temperatures=[ 25 25 ] degC  rotor_thermal_mass=50 J/K  rotor_initial_temperature=25 degC  Rm_percent_rotor=90
      settings: SourceProductName=Simscape Electronics  SourceProductBaseCode=SN
  Stepper Motor Driver : elec_lib/Actuators & Drivers/Drivers/Stepper Motor Driver  step_or_av=1  step_rate_per_volt=10 Hz/V  Venable=2.5 V  Vreverse=2.5 V  Vm=5 V  half_stepping=0
      settings: SourceProductName=Simscape Electronics  SourceProductBaseCode=SN
  Connection Port : PMIOPort  Side=Right
  wires:
  Degrees to Radians/1 -> Add/2
  PS-Simulink Converter/1 -> Add/1
  Constant1/1 -> Degrees to Radians/1
  Add/1 -> Simulink-PS Converter/1
  Fcn/1 -> Controller/1(Ref)
  In1/1 -> Fcn/1
  connections:
  Connection Port/RConn1 -- Simulink-PS Converter/RConn1
  Sensing Angle/RConn1 -- PS-Simulink Converter/LConn1
  Controller/RConn3 -- Stepper Motor Driver/LConn3
  Controller/RConn2 -- Stepper Motor Driver/LConn2
  Controller/RConn1 -- Stepper Motor Driver/LConn1
  Stepper Motor/LConn2 -- Stepper Motor Driver/RConn2
  Stepper Motor Driver/RConn3 -- Stepper Motor/LConn3
  Stepper Motor/LConn1 -- Stepper Motor Driver/RConn1 -- ERef A+/LConn1
  Solver Configuration/RConn1 -- Stepper Motor/RConn2 -- MRRef Motor/LConn1
  Shaft Free End/LConn1 -- Sensing Angle/LConn1 -- Stepper Motor/RConn1
  Stepper Motor/LConn4 -- Stepper Motor Driver/RConn4 -- ERef B-/LConn1

== system KinematicsSolverSimscape/机械臂物理模型/Joint1 ==
  note: 初始角度
  note: 初始角度
  BaseBracket_1_RIGID : Subsystem
  PS Add : fl_lib/Physical Signals/Functions/PS Add
  PS Constant : fl_lib/Physical Signals/Sources/PS Constant  constant=-pi/2
  PS Constant1 : fl_lib/Physical Signals/Sources/PS Constant  constant=-pi/2
  PS Subtract1 : fl_lib/Physical Signals/Functions/PS Subtract
      settings: SourceProductName=Simscape
  Revolute1 : sm_lib/Joints/Revolute Joint  SenseConstraintForce=off  SenseConstraintForceX=off  SenseConstraintForceY=off  SenseConstraintForceZ=off  SenseConstraintTorque=off  SenseConstraintTorqueX=off  SenseConstraintTorqueY=off  SenseConstraintTorqueZ=off  SenseTotalForce=off  SenseTotalForceX=off  SenseTotalForceY=off  SenseTotalForceZ=off  SenseTotalTorque=off  SenseTotalTorqueX=off  SenseTotalTorqueY=off  SenseTotalTorqueZ=off  CompositeWrenchDir=FollowerOnBase  CompositeWrenchFrame=BaseFrame  EquilibriumPosition=0  EquilibriumPositionUnits=rad  SpringStiffness=0  SpringStiffnessUnits=N*m/rad  DampingCoefficient=0  DampingCoefficientUnits=N*m/(rad/s)  TorqueActuationMode=ComputedTorque  MotionActuationMode=InputMotion  SensePosition=on  SenseVelocity=on  SenseAcceleration=off  SenseTorqueForce=off  PositionTargetSpecify=on  PositionTargetPriority=Low  PositionTargetValue=smiData.RevoluteJoint(2).Rz.Pos  PositionTargetValueUnits=deg  VelocityTargetSpecify=off  VelocityTargetPriority=High  VelocityTargetValue=0  VelocityTargetValueUnits=deg/s
  BaseConn : PMIOPort  Side=Left
  Motion1 : PMIOPort  Port=2  Side=Left
  q1 : PMIOPort  Port=3  Side=Right
  w1 : PMIOPort  Port=4  Side=Right
  Conn1 : PMIOPort  Port=5  Side=Right
  connections:
  BaseBracket_1_RIGID/RConn1 -- Revolute1/LConn1
  PS Add/RConn1 -- Revolute1/LConn2
  Conn1/RConn1 -- Revolute1/RConn1
  BaseBracket_1_RIGID/LConn1 -- BaseConn/RConn1
  PS Subtract1/LConn1 -- Revolute1/RConn2
  w1/RConn1 -- Revolute1/RConn3
  PS Add/LConn2 -- Motion1/RConn1
  PS Add/LConn1 -- PS Constant/RConn1
  PS Constant1/RConn1 -- PS Subtract1/LConn2
  PS Subtract1/RConn1 -- q1/RConn1

== system KinematicsSolverSimscape/机械臂物理模型/Joint2 ==
  note: 初始角度
  note: 初始角度
  Link1_2_RIGID : Subsystem
  PS Add : fl_lib/Physical Signals/Functions/PS Add
  PS Constant1 : fl_lib/Physical Signals/Sources/PS Constant  constant=-pi/2
  PS Constant2 : fl_lib/Physical Signals/Sources/PS Constant  constant=-pi/2
  PS Subtract1 : fl_lib/Physical Signals/Functions/PS Subtract
      settings: SourceProductName=Simscape
  Revolute : sm_lib/Joints/Revolute Joint  SenseConstraintForce=off  SenseConstraintForceX=off  SenseConstraintForceY=off  SenseConstraintForceZ=off  SenseConstraintTorque=off  SenseConstraintTorqueX=off  SenseConstraintTorqueY=off  SenseConstraintTorqueZ=off  SenseTotalForce=off  SenseTotalForceX=off  SenseTotalForceY=off  SenseTotalForceZ=off  SenseTotalTorque=off  SenseTotalTorqueX=off  SenseTotalTorqueY=off  SenseTotalTorqueZ=off  CompositeWrenchDir=FollowerOnBase  CompositeWrenchFrame=BaseFrame  EquilibriumPosition=0  EquilibriumPositionUnits=rad  SpringStiffness=0  SpringStiffnessUnits=N*m/rad  DampingCoefficient=0  DampingCoefficientUnits=N*m/(rad/s)  TorqueActuationMode=ComputedTorque  MotionActuationMode=InputMotion  SensePosition=on  SenseVelocity=on  SenseAcceleration=off  SenseTorqueForce=off  PositionTargetSpecify=on  PositionTargetPriority=Low  PositionTargetValue=smiData.RevoluteJoint(1).Rz.Pos  PositionTargetValueUnits=deg  VelocityTargetSpecify=off  VelocityTargetPriority=High  VelocityTargetValue=0  VelocityTargetValueUnits=deg/s
  Conn1 : PMIOPort  Side=Left
  q2 : PMIOPort  Port=2  Side=Right
  Motion2 : PMIOPort  Port=3  Side=Left
  w2 : PMIOPort  Port=4  Side=Right
  Conn2 : PMIOPort  Port=5  Side=Right
  connections:
  PS Add/LConn2 -- Motion2/RConn1
  Link1_2_RIGID/LConn1 -- Conn1/RConn1
  Link1_2_RIGID/RConn1 -- Revolute/LConn1
  Conn2/RConn1 -- Revolute/RConn1
  Revolute/RConn2 -- PS Subtract1/LConn1
  Revolute/RConn3 -- w2/RConn1
  PS Constant1/RConn1 -- PS Add/LConn1
  PS Add/RConn1 -- Revolute/LConn2
  PS Subtract1/RConn1 -- q2/RConn1
  PS Constant2/RConn1 -- PS Subtract1/LConn2

== system KinematicsSolverSimscape/机械臂物理模型/Joint3 ==
  note: 初始角度
  note: 初始角度
  Link2_2_RIGID : Subsystem
  PS Add : fl_lib/Physical Signals/Functions/PS Add
  PS Constant1 : fl_lib/Physical Signals/Sources/PS Constant  constant=0
  PS Constant2 : fl_lib/Physical Signals/Sources/PS Constant  constant=0
  PS Subtract1 : fl_lib/Physical Signals/Functions/PS Subtract
      settings: SourceProductName=Simscape
  Revolute2 : sm_lib/Joints/Revolute Joint  SenseConstraintForce=off  SenseConstraintForceX=off  SenseConstraintForceY=off  SenseConstraintForceZ=off  SenseConstraintTorque=off  SenseConstraintTorqueX=off  SenseConstraintTorqueY=off  SenseConstraintTorqueZ=off  SenseTotalForce=off  SenseTotalForceX=off  SenseTotalForceY=off  SenseTotalForceZ=off  SenseTotalTorque=off  SenseTotalTorqueX=off  SenseTotalTorqueY=off  SenseTotalTorqueZ=off  CompositeWrenchDir=FollowerOnBase  CompositeWrenchFrame=BaseFrame  EquilibriumPosition=0  EquilibriumPositionUnits=rad  SpringStiffness=0  SpringStiffnessUnits=N*m/rad  DampingCoefficient=0  DampingCoefficientUnits=N*m/(rad/s)  TorqueActuationMode=ComputedTorque  MotionActuationMode=InputMotion  SensePosition=on  SenseVelocity=on  SenseAcceleration=off  SenseTorqueForce=off  PositionTargetSpecify=on  PositionTargetPriority=Low  PositionTargetValue=smiData.RevoluteJoint(3).Rz.Pos  PositionTargetValueUnits=deg  VelocityTargetSpecify=off  VelocityTargetPriority=High  VelocityTargetValue=0  VelocityTargetValueUnits=deg/s
  Conn2 : PMIOPort  Side=Left
  Motion2 : PMIOPort  Port=2  Side=Left
  q3 : PMIOPort  Port=3  Side=Right
  w3 : PMIOPort  Port=4  Side=Right
  Conn3 : PMIOPort  Port=5  Side=Right
  connections:
  Link2_2_RIGID/RConn1 -- Revolute2/LConn1
  Link2_2_RIGID/LConn1 -- Conn2/RConn1
  PS Add/RConn1 -- Revolute2/LConn2
  PS Add/LConn1 -- PS Constant1/RConn1
  Conn3/RConn1 -- Revolute2/RConn1
  PS Constant2/RConn1 -- PS Subtract1/LConn2
  PS Subtract1/RConn1 -- q3/RConn1
  PS Subtract1/LConn1 -- Revolute2/RConn2
  w3/RConn1 -- Revolute2/RConn3
  Motion2/RConn1 -- PS Add/LConn2

== system KinematicsSolverSimscape/机械臂物理模型/Joint4 ==
  note: 初始角度
  note: 初始角度
  Link3_1_RIGID : Subsystem
  PS Add : fl_lib/Physical Signals/Functions/PS Add
  PS Constant1 : fl_lib/Physical Signals/Sources/PS Constant  constant=0
  PS Constant2 : fl_lib/Physical Signals/Sources/PS Constant  constant=0
  PS Subtract1 : fl_lib/Physical Signals/Functions/PS Subtract
      settings: SourceProductName=Simscape
  Revolute3 : sm_lib/Joints/Revolute Joint  SenseConstraintForce=off  SenseConstraintForceX=off  SenseConstraintForceY=off  SenseConstraintForceZ=off  SenseConstraintTorque=off  SenseConstraintTorqueX=off  SenseConstraintTorqueY=off  SenseConstraintTorqueZ=off  SenseTotalForce=off  SenseTotalForceX=off  SenseTotalForceY=off  SenseTotalForceZ=off  SenseTotalTorque=off  SenseTotalTorqueX=off  SenseTotalTorqueY=off  SenseTotalTorqueZ=off  CompositeWrenchDir=FollowerOnBase  CompositeWrenchFrame=BaseFrame  EquilibriumPosition=0  EquilibriumPositionUnits=rad  SpringStiffness=0  SpringStiffnessUnits=N*m/rad  DampingCoefficient=0  DampingCoefficientUnits=N*m/(rad/s)  TorqueActuationMode=ComputedTorque  MotionActuationMode=InputMotion  SensePosition=on  SenseVelocity=on  SenseAcceleration=off  SenseTorqueForce=off  PositionTargetSpecify=on  PositionTargetPriority=Low  PositionTargetValue=smiData.RevoluteJoint(4).Rz.Pos  PositionTargetValueUnits=deg  VelocityTargetSpecify=off  VelocityTargetPriority=High  VelocityTargetValue=0  VelocityTargetValueUnits=deg/s
  Conn3 : PMIOPort  Side=Left
  Motion4 : PMIOPort  Port=2  Side=Left
  q4 : PMIOPort  Port=3  Side=Right
  w4 : PMIOPort  Port=4  Side=Right
  Conn4 : PMIOPort  Port=5  Side=Right
  connections:
  PS Add/RConn1 -- Revolute3/LConn2
  Link3_1_RIGID/RConn1 -- Revolute3/LConn1
  Link3_1_RIGID/LConn1 -- Conn3/RConn1
  PS Subtract1/LConn1 -- Revolute3/RConn2
  PS Add/LConn2 -- Motion4/RConn1
  PS Subtract1/RConn1 -- q4/RConn1
  PS Constant2/RConn1 -- PS Subtract1/LConn2
  Conn4/RConn1 -- Revolute3/RConn1
  PS Add/LConn1 -- PS Constant1/RConn1
  w4/RConn1 -- Revolute3/RConn3

== system KinematicsSolverSimscape/机械臂物理模型/Joint5 ==
  note: 初始角度
  note: 初始角度
  Link4_1_RIGID : Subsystem
  PS Add : fl_lib/Physical Signals/Functions/PS Add
  PS Constant1 : fl_lib/Physical Signals/Sources/PS Constant  constant=pi/2
  PS Constant2 : fl_lib/Physical Signals/Sources/PS Constant  constant=pi/2
  PS Subtract1 : fl_lib/Physical Signals/Functions/PS Subtract
      settings: SourceProductName=Simscape
  Revolute5 : sm_lib/Joints/Revolute Joint  SenseConstraintForce=off  SenseConstraintForceX=off  SenseConstraintForceY=off  SenseConstraintForceZ=off  SenseConstraintTorque=off  SenseConstraintTorqueX=off  SenseConstraintTorqueY=off  SenseConstraintTorqueZ=off  SenseTotalForce=off  SenseTotalForceX=off  SenseTotalForceY=off  SenseTotalForceZ=off  SenseTotalTorque=off  SenseTotalTorqueX=off  SenseTotalTorqueY=off  SenseTotalTorqueZ=off  CompositeWrenchDir=FollowerOnBase  CompositeWrenchFrame=BaseFrame  EquilibriumPosition=0  EquilibriumPositionUnits=rad  SpringStiffness=0  SpringStiffnessUnits=N*m/rad  DampingCoefficient=0  DampingCoefficientUnits=N*m/(rad/s)  TorqueActuationMode=ComputedTorque  MotionActuationMode=InputMotion  SensePosition=on  SenseVelocity=on  SenseAcceleration=off  SenseTorqueForce=off  PositionTargetSpecify=on  PositionTargetPriority=Low  PositionTargetValue=smiData.RevoluteJoint(5).Rz.Pos  PositionTargetValueUnits=deg  VelocityTargetSpecify=off  VelocityTargetPriority=High  VelocityTargetValue=0  VelocityTargetValueUnits=deg/s
  Conn4 : PMIOPort  Side=Left
  Motion5 : PMIOPort  Port=2  Side=Left
  q5 : PMIOPort  Port=3  Side=Right
  w5 : PMIOPort  Port=4  Side=Right
  Conn5 : PMIOPort  Port=5  Side=Right
  connections:
  Link4_1_RIGID/RConn1 -- Revolute5/LConn1
  PS Add/RConn1 -- Revolute5/LConn2
  Link4_1_RIGID/LConn1 -- Conn4/RConn1
  PS Subtract1/LConn1 -- Revolute5/RConn2
  PS Add/LConn2 -- Motion5/RConn1
  PS Subtract1/RConn1 -- q5/RConn1
  PS Constant2/RConn1 -- PS Subtract1/LConn2
  Conn5/RConn1 -- Revolute5/RConn1
  PS Constant1/RConn1 -- PS Add/LConn1
  w5/RConn1 -- Revolute5/RConn3
